simulink model "openManipulatorTorqueCtrlConfig"  (R2022b)
settings: Solver=VariableStepAuto  StartTime=0.0  StopTime=20  RelTol=1e-3
PreLoadFcn:
  | openManipulatorParameters;
undefined symbols (not defined in the file): TsCtrl
libraries: OpenManipulatorLib x3, sm_lib x2, nesl_utility x1
settings Model: Creator=scastro  LastModifiedBy=Boog
settings SolverCC: AlgebraicLoopSolver=TrustRegion  DecoupledContinuousIntegration=on  MinimalZcImpactIntegration=on
settings DataIOCC: ReturnWorkspaceOutputs=off
settings DebuggingCC: UnconnectedInputMsg=warning  UnconnectedOutputMsg=warning  UnconnectedLineMsg=warning  SFMachineParentedDataDiag=warning  ArithmeticOperatorsInVariantConditions=warning
settings ModelReferenceCC: EnableRefExpFcnMdlSchedulingChecks=on
settings SFSimCC: SimUseLocalCustomCode=off  CustomCodeUndefinedFunction=UseInterfaceOnly
settings RTWCC: RTWUseLocalCustomCode=off
settings ExplorerConfigSet: InternalSimMechanicsExplorerSettings="<ExplorerConfiguration><canonicalview>default</canonicalview><AnimationSetting><BasePlaybackSpeed>1.0</BasePlaybackSpeed><PlaybackSpeedFactor>1.0</PlaybackSpeedFactor></AnimationSetting><TilePanel><TileInfo><Tiles Columns=\"1\" Count=\"1\" Rows=\"1\"><Column Weight=\"1\"/><Row Weight=\"1\"/><Tile Height=\"1\" Width=\"1\" X=\"0\" Y=\"0\"/></Tiles></TileInfo><SceneInfo><SceneViewer><BGColor><R>0.60000002384185791</R><G>0.60000002384185791</G><B>0.60000002384185791</B></BGColor><Camera><DoPerspective>off</DoPerspective><Position><X>0.428752942017998073</X><Y>-0.712150369953937545</Y><Z>0.628314823463847372</Z></Position><Center><X>0.0455703138120887447</X><Y>0.0802507835591396851</Y><Z>0.153687090021758288</Z></Center><Up><X>-0.128866037345358619</X><Y>0.462960972240881619</Y><Z>0.876961049648547597</Z></Up><ViewLimDist>1</ViewLimDist><YLim>0.579070269035580121</YLim><XLim>0.64437894599448009</XLim></Camera></SceneViewer></SceneInfo></TilePanel><MechEditorPanel><Cameras/><GfxPanelCameraMap/><VideoCreator><PlaybackSpeedRatio>1.0</PlaybackSpeedRatio><FrameRate>30</FrameRate><VideoFormat>Motion JPEG AVI</VideoFormat><FrameSize>auto</FrameSize></VideoCreator></MechEditorPanel></ExplorerConfiguration>"

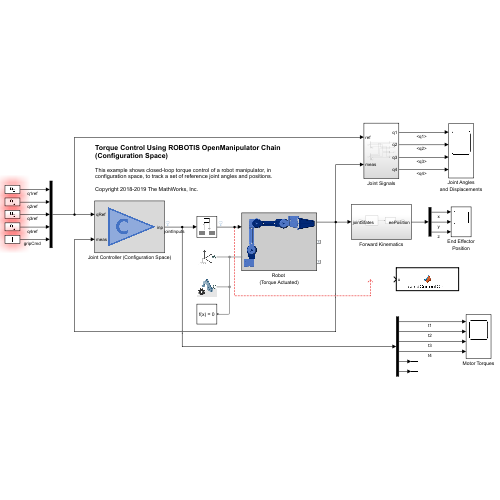
[thumbnail: Simulink's stored preview of the top-level diagram]
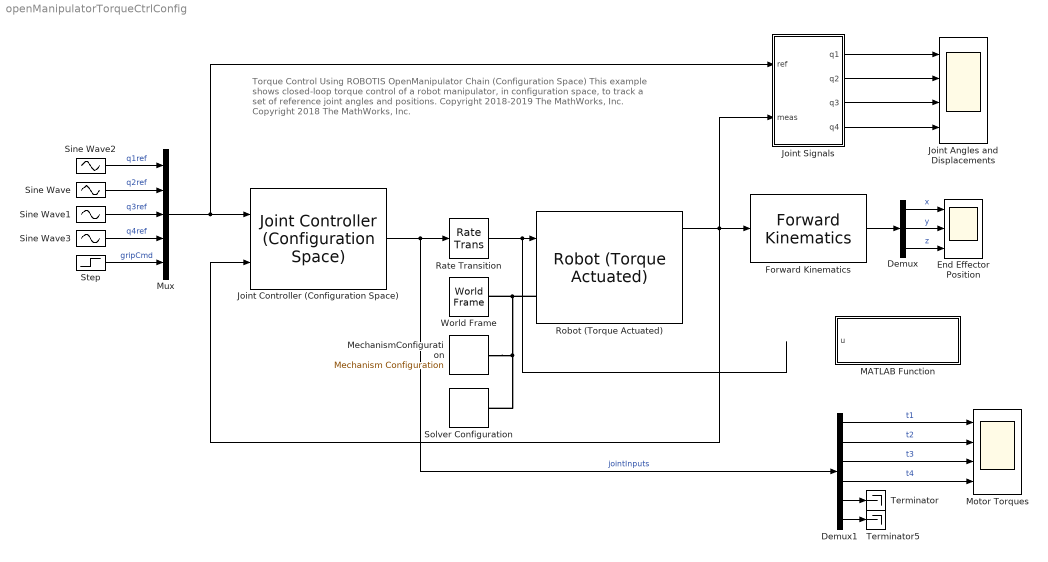
== system openManipulatorTorqueCtrlConfig ==
  note: Torque Control Using ROBOTIS OpenManipulator Chain (Configuration Space)
      |
      | This example shows closed-loop torque control of a robot manipulator, in configuration space, to track a set of reference joint angles and positions.
      |
      | Copyright 2018-2019 The MathWorks, Inc.
      |
      | Copyright 2018 The MathWorks, Inc.
  Demux : Demux  Outputs=3
  Demux1 : Demux  Outputs=6
  End Effector Position : Scope  NumInputPorts=3
  Forward Kinematics : OpenManipulatorLib/Forward Kinematics  SystemSampleTime=-1  VariantActivationTime=update diagram  Latency=0  AutoFrameSizeCalculation=off
  Joint Angles and Displacements : Scope  NumInputPorts=4
  Joint Controller (Configuration Space) : OpenManipulatorLib/Joint Controller (Configuration Space)  SystemSampleTime=-1  VariantControl=ctrlType==1  VariantActivationTime=update diagram  Latency=0  AutoFrameSizeCalculation=off
  Joint Signals : Subsystem
  MATLAB Function : MATLAB Function  TreatAsAtomicUnit=on
  MechanismConfiguration : sm_lib/Utilities/Mechanism Configuration  UniformGravity=Constant  GravityVector=[0 0 -9.80665]  GravityUnits=m/s^2  LinearizationDelta=0.001  JointModeTransitionNonlinearIterations=2
  Motor Torques : Scope  NumInputPorts=4
  Mux : Mux  Inputs=5
  Rate Transition : RateTransition
  Robot (Torque Actuated) : OpenManipulatorLib/Robot  (Torque Actuated)  SystemSampleTime=-1  VariantActivationTime=update diagram  Latency=0  AutoFrameSizeCalculation=off
  Sine Wave : Sin  Amplitude=pi/4  Frequency=0.6  SampleTime=TsCtrl
  Sine Wave1 : Sin  Amplitude=pi/4  Frequency=1.5  SampleTime=TsCtrl
  Sine Wave2 : Sin  Amplitude=2*pi/3  Frequency=0.4  SampleTime=TsCtrl
  Sine Wave3 : Sin  Amplitude=pi/3  SampleTime=TsCtrl
  Solver Configuration : nesl_utility/Solver Configuration  PhysicalDomain=network_engine_domain  SubClassName=solver  LeftPortType=input  RightPortType=generic  Tones=[]  Harmonics=[]  SimulateNoise=off  Profile=off  UseLocalSampling=off  EnableSwitchedLinearOptims=on  FrequencyDomain=off  UseCCode=off  RelTol=0.001  AbsTol=1e-06  MinStep=1e-09  ToWorkspace=off  RevertToSquareIcSolve=off  NumHomotopyIterations=100  PhasorMode=off  PhasorModeNumHarmonics=1  ConsistencySolver=NEWTON_FTOL  IndexReductionMethod=DerivativeReplacement  DoDC=off  ResidualTolerance=1e-09  ConsistencyTolSource=GLOBAL  ConsistencyAbsTol=0.001  ConsistencyRelTol=0.001  ConsistencyTolFactor=0.001  UseLocalSolver=off  LocalSolverChoice=NE_BACKWARD_EULER_ADVANCER  ResolveIndetEquations=on  FunctionEvalNumThread=1  LocalSolverSampleTime=0.001  DoFixedCost=off  MaxNonlinIter=3  MaxModeIter=2  ComputeImpulses=off  ImpulseIterations=2  LinearAlgebra=Sparse  LinearAlgebraNumThread=0  EquationFormulation=NE_TIME_EF  DelaysMemoryBudget=1024  AutomaticFiltering=on  FilteringTimeConstant=0.001  PartitionStorageMethod=AS_NEEDED  PartitionMemoryBudget=1024  PartitionMethod=FAST
  Step : Step  Time=5  SampleTime=TsCtrl
  Terminator : Terminator
  Terminator5 : Terminator
  World Frame : sm_lib/Frames and Transforms/World Frame
  wires:
  Robot (Torque Actuated)/1 -> Joint Controller (Configuration Space)/2, Forward Kinematics/1, Joint Signals/2(meas)
  Sine Wave/1 -> Mux/2  "q2ref"
  Sine Wave1/1 -> Mux/3  "q3ref"
  Sine Wave2/1 -> Mux/1  "q1ref"
  Rate Transition/1 -> Robot (Torque Actuated)/1
  Mux/1 -> Joint Controller (Configuration Space)/1, Joint Signals/1(ref)
  Joint Signals/1(q1) -> Joint Angles and Displacements/1
  Joint Signals/2(q2) -> Joint Angles and Displacements/2
  Joint Signals/3(q3) -> Joint Angles and Displacements/3
  Joint Signals/4(q4) -> Joint Angles and Displacements/4
  Sine Wave3/1 -> Mux/4  "q4ref"
  Step/1 -> Mux/5  "gripCmd"
  Joint Controller (Configuration Space)/1 -> Demux1/1, Rate Transition/1  "jointInputs"
  Forward Kinematics/1 -> Demux/1
  Demux/1 -> End Effector Position/1  "x"
  Demux/2 -> End Effector Position/2  "y"
  Demux/3 -> End Effector Position/3  "z"
  Demux1/5 -> Terminator/1
  Demux1/4 -> Motor Torques/4  "t4"
  Demux1/3 -> Motor Torques/3  "t3"
  Demux1/2 -> Motor Torques/2  "t2"
  Demux1/1 -> Motor Torques/1  "t1"
  Demux1/6 -> Terminator5/1
  connections:
  Robot (Torque Actuated)/LConn1 -- Solver Configuration/RConn1 -- MechanismConfiguration/RConn1 -- World Frame/RConn1

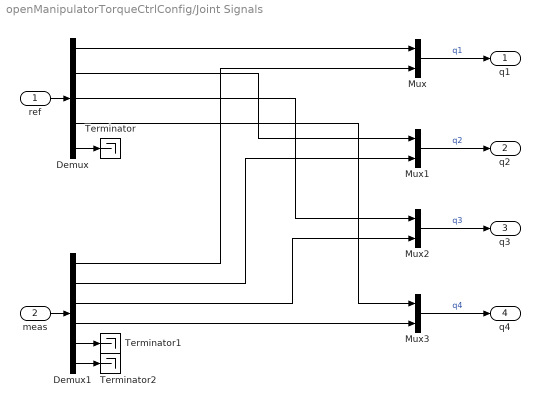
== system openManipulatorTorqueCtrlConfig/Joint Signals ==
  ref : Inport
  meas : Inport  Port=2
  Demux : Demux  Outputs=5
  Demux1 : Demux  Outputs=6
  Mux{,1..3} (4 alike) : Mux  Inputs=2
  Terminator : Terminator
  Terminator1 : Terminator
  Terminator2 : Terminator
  q1 : Outport  VectorParamsAs1DForOutWhenUnconnected=off
  q2 : Outport  Port=2  VectorParamsAs1DForOutWhenUnconnected=off
  q3 : Outport  Port=3  VectorParamsAs1DForOutWhenUnconnected=off
  q4 : Outport  Port=4  VectorParamsAs1DForOutWhenUnconnected=off
  wires:
  Mux2/1 -> q3/1  "q3"
  ref/1 -> Demux/1
  Mux3/1 -> q4/1  "q4"
  Mux/1 -> q1/1  "q1"
  meas/1 -> Demux1/1
  Demux/1 -> Mux/1
  Demux1/1 -> Mux/2
  Mux1/1 -> q2/1  "q2"
  Demux/2 -> Mux1/1
  Demux1/2 -> Mux1/2
  Demux/3 -> Mux2/1
  Demux1/3 -> Mux2/2
  Demux1/4 -> Mux3/2
  Demux/4 -> Mux3/1
  Demux/5 -> Terminator/1
  Demux1/5 -> Terminator1/1
  Demux1/6 -> Terminator2/1

== matlab function openManipulatorTorqueCtrlConfig/MATLAB Function ==
  data: u input
function sendCurrentOne(u)

    % 1.5A / 1.6 N-m
    
    % 0.9375 A/N-m
    
    % Current in Amps = 0.9375 * t[N-m]

    % Current in mA = Current in Amps * 1000

    % Current in Data = Current in mA / 2.69

    current_A = 0.9375 .* u;
    
    current_data = current_A .* 1000 ./ 2.69;
    
    % Write goal current
    write2ByteTxRx(port_num, PROTOCOL_VERSION, DXL_ID, ADDR_GOAL_CURRENT, typecast(int16(current_data(1)), 'uint16'));    % typecast(int32(-2000), 'uint32')
    dxl_comm_result = getLastTxRxResult(port_num, PROTOCOL_VERSION);
    dxl_error = getLastRxPacketError(port_num, PROTOCOL_VERSION);
    if dxl_comm_result ~= COMM_SUCCESS
        fprintf('%s\n', getTxRxResult(PROTOCOL_VERSION, dxl_comm_result));
    elseif dxl_error ~= 0
        fprintf('%s\n', getRxPacketError(PROTOCOL_VERSION, dxl_error));
    end  
end
